simulink library "roshelperlib"  (R2024a)
settings: Solver=VariableStepAuto  StartTime=0.0  StopTime=10.0  RelTol=1e-3
values from neighbouring files (symbols this model uses):
  data = rand(prod(dims),1)    [bufferAssignTest.m]
  isVarsize = ws.get('isVarsize')    [extractmulticallbacks.m]    (also in gendatacallbacks.m = varsizeDims; rospubcallbacks.m = matlab.lang.OnOffSwitchState(commonmaskutils.getWSValue('isV; rossubcallbacks.m)
  varsize = false    [visualizeScene.m]
undefined symbols (not defined in the file or in its folder): data_SL_Info, layout, stride, x, y, z
libraries: ros2lib x4, $bdroot x2
settings Model: Creator=cstabile  LastModifiedBy=cstabile

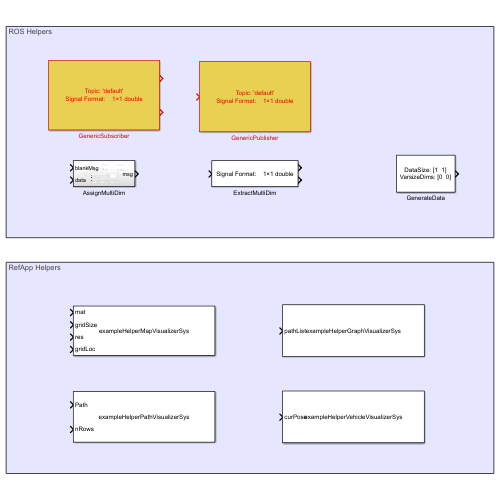
[thumbnail: Simulink's stored preview of the top-level diagram]
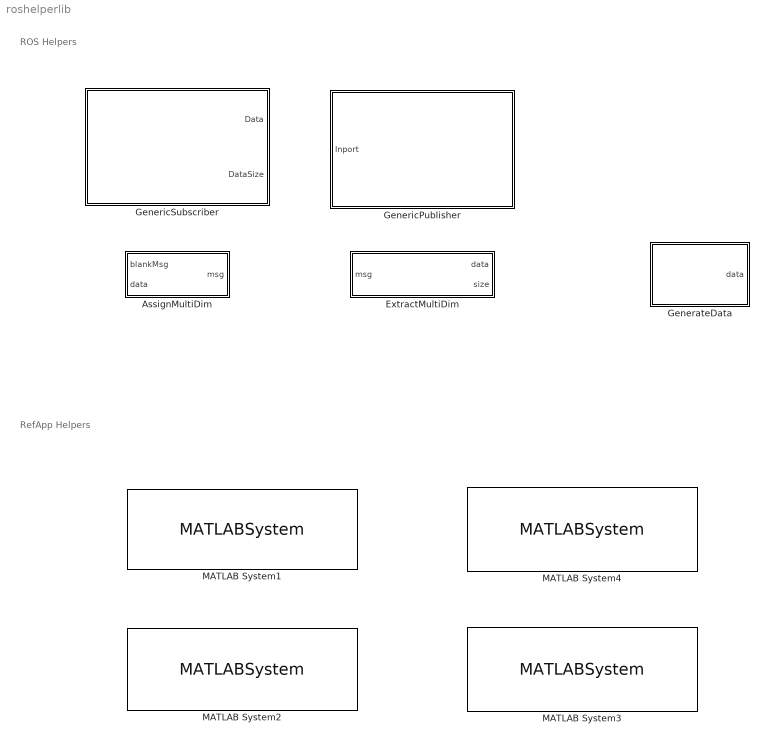
== system roshelperlib ==
  note: ROS Helpers
  note: RefApp Helpers
  AssignMultiDim : Subsystem
  ExtractMultiDim : Subsystem  mask{userDataType=double, dims=[1 1], isVarsize=off, varsizeDims=[], returnFixedTF=off}
      mask prompts: userDataType "DataType"; dims "MaxDimensions"; isVarsize "IsVarsize?"; returnFixedTF "ReturnFixed?"
      mask Display:
      | userDataType = char(get_param(gcb,'userDataType'));
      | isVarsize = matlab.lang.OnOffSwitchState(get_param(gcb,'isVarsize'));
      | dims = eval(get_param(gcb,'dims'));
      | vDims = eval(get_param(gcb,'varsizeDims'));
      | returnFixedTF = matlab.lang.OnOffSwitchState(get_param(gcb,'returnFixedTF'));
      | 
      | data = zeros(0,userDataType);
      | if isVarsize && returnFixedTF == 0 && any(vDims)
      |     type = coder.typeof(data,dims,vDims);
      | else
      |     type = coder.typeof(data,dims);
      | end
      | strs = string(splitlines(formattedDisplayText(type)));
      | dataStr = strs(2);
      | 
      | dispStrings(1) = string(['Signal Format' ': ' char(dataStr)]);
      | if isVarsize
      |     dispStrings(2) = string(['VarsizeDimensions' ': ' '[' num2str(vDims) ']']);
      | end
      | 
      | disp(dispStrings);
  GenerateData : Subsystem  mask{dataSize=[1 1], varsizeDims=[]}
      mask Display:
      | dataSize = eval(get_param(gcb,'dataSize'));
      | mask = Simulink.Mask.get(gcb);
      | vars = mask.getWorkspaceVariables;
      | isVarsize = vars(arrayfun(@(x)isequal(x.Name,'isVarsize'),vars)).Value;
      | 
      | dispStr(1) = "DataSize: " + "[" + num2str(dataSize) + "]";
      | dispStr(2) = "VarsizeDims: " + "[" + num2str(isVarsize) + "]";
      | disp(dispStr);
  GenericPublisher : Subsystem  mask{userDataType=double, dims=[1 1], topicName='default', isVarsize=off, varsizeDims=[1 0]}
      mask prompts: userDataType "Type"; dims "MaxDimension"; isVarsize "IsVarsize?"; varsizeDims "VszDims"
      mask Display:
      | userDataType = char(get_param(gcb,'userDataType'));
      | topicName = char(get_param(gcb,'topicName'));
      | isVarsize = matlab.lang.OnOffSwitchState(get_param(gcb,'isVarsize'));
      | dims = eval(get_param(gcb,'dims'));
      | vDims = eval(get_param(gcb,'varsizeDims'));
      | 
      | data = zeros(0,userDataType);
      | if isVarsize && any(vDims)
      |     type = coder.typeof(data,dims,vDims);
      | else
      |     type = coder.typeof(data,dims);
      | end
      | strs = string(splitlines(formattedDisplayText(type)));
      | dataStr = strs(2);
      | 
      | dispStrings(1) = string(['Topic' ': ' char(topicName)]);
      | dispStrings(2) = string(['Signal Format' ': ' char(dataStr)]);
      | % dispStrings(3) = string(['VarsizeDimensions' ': ' '[' num2str(vDims) ']']);
      | disp(dispStrings);
  GenericSubscriber : Subsystem  mask{userDataType=double, dims=[1 1], topicName='default', isVarsize=off, varsizeDims=[1 0], returnFixedTF=off}
      mask prompts: userDataType "Type"; dims "MaxDimension"; isVarsize "IsVarsize?"; varsizeDims "VszDims"; returnFixedTF "ReturnFixed"
      mask Display:
      | userDataType = char(get_param(gcb,'userDataType'));
      | topicName = char(get_param(gcb,'topicName'));
      | isVarsize = matlab.lang.OnOffSwitchState(get_param(gcb,'isVarsize'));
      | dims = eval(get_param(gcb,'dims'));
      | vDims = eval(get_param(gcb,'varsizeDims'));
      | returnFixedTF = matlab.lang.OnOffSwitchState(get_param(gcb,'returnFixedTF'));
      | 
      | data = zeros(0,userDataType);
      | if isVarsize && returnFixedTF == 0 && any(vDims)
      |     type = coder.typeof(data,dims,vDims);
      | else
      |     type = coder.typeof(data,dims);
      | end
      | strs = string(splitlines(formattedDisplayText(type)));
      | dataStr = strs(2);
      | 
      | dispStrings(1) = string(['Topic' ': ' char(topicName)]);
      | dispStrings(2) = string(['Signal Format' ': ' char(dataStr)]);
      | if isVarsize
      |     dispStrings(3) = string(['VarsizeDimensions' ': ' '[' num2str(vDims) ']']);
      | end
      | disp(dispStrings);
  MATLAB System1 : MATLABSystem  System=exampleHelperMapVisualizerSys  MapType=SDF  DisplayVisual=on  SimulateUsing=Interpreted execution
      mask Type: exampleHelperMapVisualizerSys
      mask Display:
      | disp('exampleHelperMapVisualizerSys');
      | port_label('input',1,'mat');
      | port_label('input',2,'gridSize');
      | port_label('input',3,'res');
      | port_label('input',4,'gridLoc');
  MATLAB System2 : MATLABSystem  System=exampleHelperPathVisualizerSys  VisualizationParameters={'k-'}  PlotType=Line  DisplayVisual=on  SimulateUsing=Interpreted execution
      mask Type: exampleHelperPathVisualizerSys
      mask Display:
      | disp('exampleHelperPathVisualizerSys');
      | port_label('input',1,'Path');
      | port_label('input',2,'nRows');
  MATLAB System3 : MATLABSystem  System=exampleHelperVehicleVisualizerSys  NumCircles=3  Length=4  Width=2  DisplayVisual=on  SimulateUsing=Interpreted execution
      mask Type: exampleHelperVehicleVisualizerSys
      mask Display:
      | disp('exampleHelperVehicleVisualizerSys');
      | port_label('input',1,'curPose');
  MATLAB System4 : MATLABSystem  System=exampleHelperGraphVisualizerSys  NodeColor=r  EdgeColor=r  LineStyle=-  GraphSpec=cell(1,0)  NetworkColor=b  NetworkStyle=:  NetworkSpec=cell(1,0)  MaxEdgeElem=Inf  NetworkAlpha=1  EdgeAlpha=1  DisplayVisual=on  SimulateUsing=Interpreted execution
      mask Type: exampleHelperGraphVisualizerSys
      mask Display:
      | disp('exampleHelperGraphVisualizerSys');
      | port_label('input',1,'pathList');

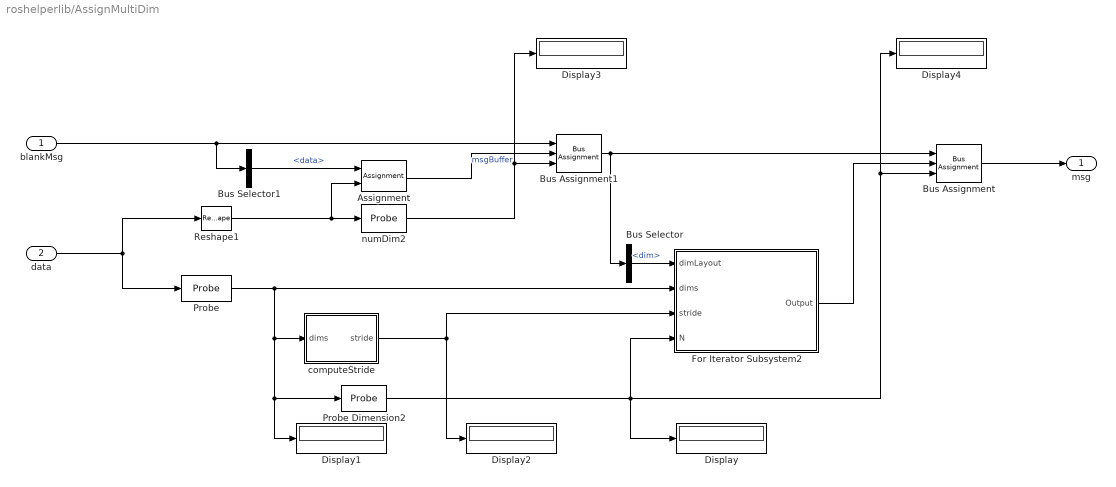
== system roshelperlib/AssignMultiDim ==
  blankMsg : Inport
  data : Inport  Port=2
  Assignment : Assignment  DiagnosticForDimensions=Warning  IndexOptions=Starting index (dialog)  Indices=1  OutputSizes=1
  Bus Assignment : BusAssignment  AssignedSignals=layout.dim,layout.dim_SL_Info.CurrentLength
  Bus Assignment1 : BusAssignment  AssignedSignals=data,data_SL_Info.CurrentLength
  Bus Selector : BusSelector  OutputSignals=layout.dim
  Bus Selector1 : BusSelector  OutputSignals=data
  Display{,1..4} (5 alike) : Display
  For Iterator Subsystem2 : Subsystem  TreatAsAtomicUnit=on
  Probe : Probe  ProbeWidth=off  ProbeSampleTime=off  ProbeComplexSignal=off  ProbeSignalDimensions=on
  Probe Dimension2 : Probe  ProbeWidth=off  ProbeSampleTime=off  ProbeComplexSignal=off  ProbeSignalDimensions=on  ProbeWidthDataType=uint32  ProbeDimensionsDataType=uint32
  Reshape1 : Reshape
  computeStride : MATLAB Function  TreatAsAtomicUnit=on
  numDim2 : Probe  ProbeSampleTime=off  ProbeComplexSignal=off  ProbeWidthDataType=uint32
  msg : Outport
  wires:
  Bus Selector1/1 -> Assignment/1  "<data>"
  Bus Selector/1 -> For Iterator Subsystem2/1(dimLayout)  "<dim>"
  Assignment/1 -> Bus Assignment1/2  "msgBuffer"
  Bus Assignment1/1 -> Bus Selector/1, Bus Assignment/1
  Probe Dimension2/1 -> For Iterator Subsystem2/4(N), Display/1, Display4/1, Bus Assignment/3
  computeStride/1(stride) -> For Iterator Subsystem2/3(stride), Display2/1
  For Iterator Subsystem2/1(Output) -> Bus Assignment/2
  blankMsg/1 -> Bus Selector1/1, Bus Assignment1/1
  Bus Assignment/1 -> msg/1
  Probe/1 -> For Iterator Subsystem2/2(dims), Probe Dimension2/1, Display1/1, computeStride/1(dims)
  numDim2/1 -> Display3/1, Bus Assignment1/3
  Reshape1/1 -> numDim2/1, Assignment/2
  data/1 -> Probe/1, Reshape1/1

== system roshelperlib/ExtractMultiDim ==
  msg : Inport
  FixedOrVarOutput : Subsystem  Variant=on  VariantControl=Subsystem
  data : Outport
  size : Outport  Port=2
  wires:
  msg/1 -> FixedOrVarOutput/1(msg)
  FixedOrVarOutput/1(data) -> data/1
  FixedOrVarOutput/2(size) -> size/1

== system roshelperlib/GenerateData ==
  Subsystem : Subsystem  Variant=on  VariantControl=Subsystem
  data : Outport
  wires:
  Subsystem/1(data) -> data/1

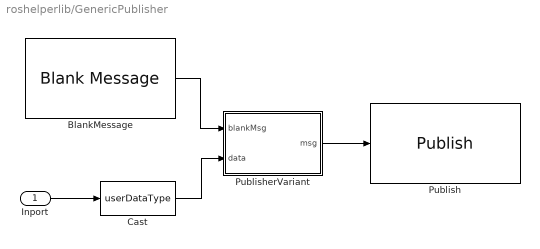
== system roshelperlib/GenericPublisher ==
  Inport : Inport
  BlankMessage : ros2lib/Blank Message  VariantControl=Choice_1  messageClass=Message  entityType=std_msgs/Float64  messageType=std_msgs/Float64  SampleTime=inf
  Cast : DataTypeConversion  OutDataTypeStr=userDataType  SaturateOnIntegerOverflow=off  RndMeth=Floor
  Publish : ros2lib/Publish  topicSource=Select from ROS network  topic=/default  messageType=std_msgs/Float64  QOSHistory=Keep last  QOSDepth=1  QOSReliability=Reliable  QOSDurability=Volatile  QOSDeadline=Inf  QOSLifespan=Inf  QOSLiveliness=Automatic  QOSLeaseDuration=Inf  QOSAvoidROSNamespaceConventions=off
  PublisherVariant : Subsystem  Variant=on  VariantControl=useFixedTF==0
  wires:
  Inport/1 -> Cast/1
  Cast/1 -> PublisherVariant/2(data)
  BlankMessage/1 -> PublisherVariant/1(blankMsg)
  PublisherVariant/1(msg) -> Publish/1

== system roshelperlib/GenericSubscriber ==
  SubscriberVariant : Subsystem  Variant=on  VariantControl=useFixedTF==0
  Data : Outport
  DataSize : Outport  Port=2
  wires:
  SubscriberVariant/2(Output1) -> DataSize/1
  SubscriberVariant/1(Output) -> Data/1

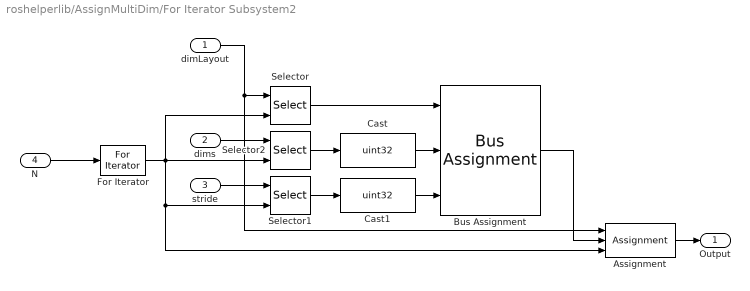
== system roshelperlib/AssignMultiDim/For Iterator Subsystem2 ==
  dimLayout : Inport
  dims : Inport  Port=2
  stride : Inport  Port=3
  N : Inport  Port=4
  Assignment : Assignment  DiagnosticForDimensions=Warning  IndexOptions=Index vector (port)  Indices=1  OutputSizes=1
  Bus Assignment : BusAssignment  AssignedSignals=size,stride
  Cast : DataTypeConversion  OutDataTypeStr=uint32  SaturateOnIntegerOverflow=off  RndMeth=Floor
  Cast1 : DataTypeConversion  OutDataTypeStr=uint32  SaturateOnIntegerOverflow=off  RndMeth=Floor
  For Iterator : ForIterator  IterationSource=external  IterationLimit=16
  Selector : Selector  InputPortWidth=16  IndexOptions=Index vector (port)  Indices=[1 3]  OutputSizes=1
  Selector1 : Selector  IndexOptions=Index vector (port)  Indices=[1 3]  OutputSizes=1
  Selector2 : Selector  IndexOptions=Index vector (port)  Indices=[1 3]  OutputSizes=1
  Output : Outport
  wires:
  stride/1 -> Selector1/1
  dims/1 -> Selector2/1
  Bus Assignment/1 -> Assignment/2
  dimLayout/1 -> Assignment/1, Selector/1
  Selector/1 -> Bus Assignment/1
  For Iterator/1 -> Selector2/2, Selector1/2, Assignment/3, Selector/2
  N/1 -> For Iterator/1
  Selector1/1 -> Cast1/1
  Selector2/1 -> Cast/1
  Assignment/1 -> Output/1
  Cast/1 -> Bus Assignment/2
  Cast1/1 -> Bus Assignment/3

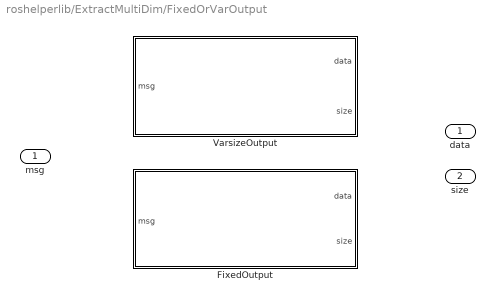
== system roshelperlib/ExtractMultiDim/FixedOrVarOutput ==
  msg : Inport
  FixedOutput : Subsystem  VariantControl=outputIsFixedTF==1
  VarsizeOutput : Subsystem  VariantControl=outputIsFixedTF==0
  data : Outport
  size : Outport  Port=2

== system roshelperlib/GenerateData/Subsystem ==
  Fixed : Subsystem  VariantControl=variantFixedTF == 1
  Varsize : Subsystem  VariantControl=variantFixedTF == 0
  data : Outport

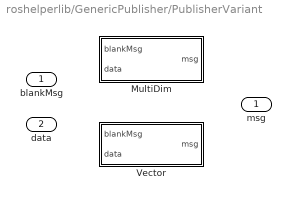
== system roshelperlib/GenericPublisher/PublisherVariant ==
  blankMsg : Inport
  data : Inport  Port=2
  MultiDim : Subsystem  VariantControl=useVarsizeTF==1
  Vector : Subsystem  VariantControl=useVarsizeTF==0
  msg : Outport

== system roshelperlib/GenericSubscriber/SubscriberVariant ==
  MultiDim : Subsystem  VariantControl=useMultiDimTF==1
  Vector : Subsystem  VariantControl=useMultiDimTF==0
  Output : Outport
  Output1 : Outport  Port=2

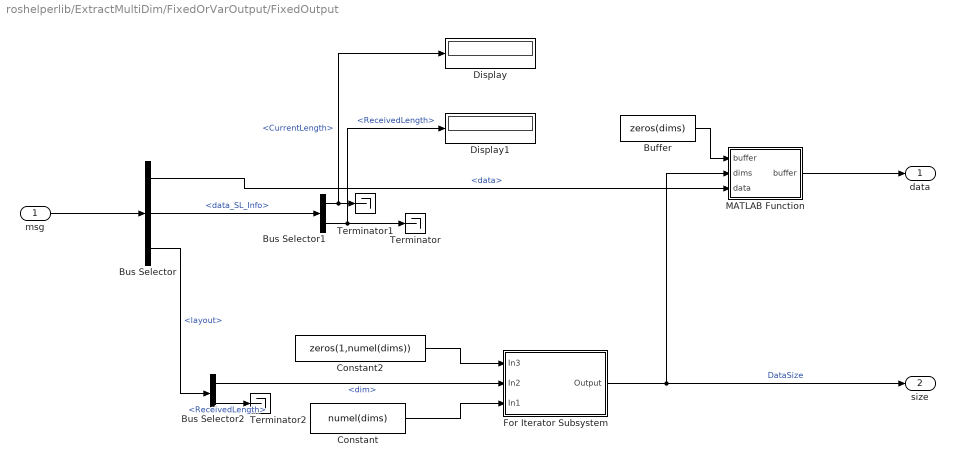
== system roshelperlib/ExtractMultiDim/FixedOrVarOutput/FixedOutput ==
  msg : Inport
  Buffer : Constant  Value=zeros(dims)  OutDataTypeStr=userDataType
  Bus Selector : BusSelector  OutputSignals=data,data_SL_Info,layout
  Bus Selector1 : BusSelector  OutputSignals=CurrentLength,ReceivedLength
  Bus Selector2 : BusSelector  OutputSignals=dim,dim_SL_Info.ReceivedLength
  Constant : Constant  Value=numel(dims)
  Constant2 : Constant  Value=zeros(1,numel(dims))  VectorParams1D=off
  Display : Display
  Display1 : Display
  For Iterator Subsystem : Subsystem  TreatAsAtomicUnit=on
  MATLAB Function : MATLAB Function  TreatAsAtomicUnit=on
  Terminator : Terminator
  Terminator1 : Terminator
  Terminator2 : Terminator
  data : Outport
  size : Outport  Port=2
  wires:
  Bus Selector/1 -> MATLAB Function/3(data)  "<data>"
  Bus Selector2/1 -> For Iterator Subsystem/2(In2)  "<dim>"
  For Iterator Subsystem/1(Output) -> MATLAB Function/2(dims), size/1  "DataSize"
  Bus Selector/3 -> Bus Selector2/1  "<layout>"
  Bus Selector2/2 -> Terminator2/1  "<ReceivedLength>"
  Bus Selector1/2 -> Terminator/1, Display1/1  "<ReceivedLength>"
  Bus Selector1/1 -> Terminator1/1, Display/1  "<CurrentLength>"
  MATLAB Function/1(buffer) -> data/1
  Buffer/1 -> MATLAB Function/1("buffer ")
  Constant2/1 -> For Iterator Subsystem/1(In3)
  Bus Selector/2 -> Bus Selector1/1  "<data_SL_Info>"
  msg/1 -> Bus Selector/1
  Constant/1 -> For Iterator Subsystem/3(In1)

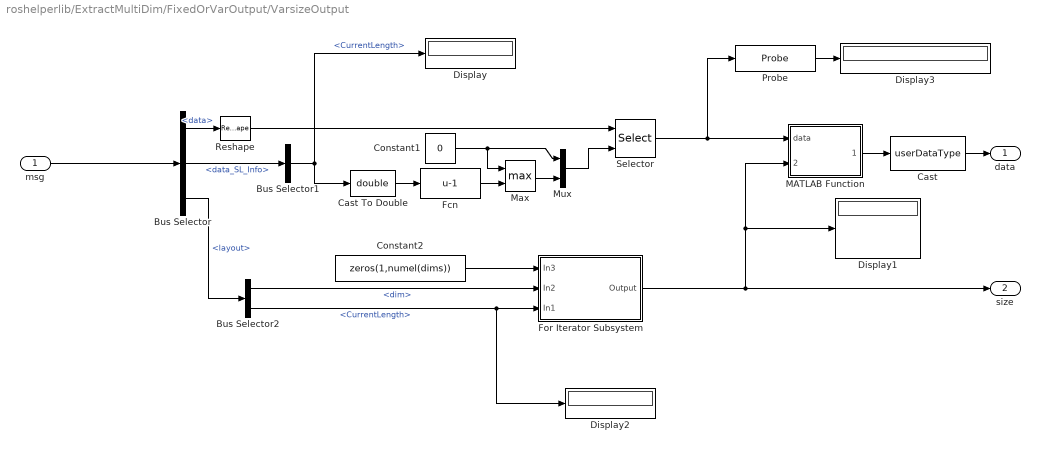
== system roshelperlib/ExtractMultiDim/FixedOrVarOutput/VarsizeOutput ==
  msg : Inport
  Bus Selector : BusSelector  OutputSignals=data,data_SL_Info,layout
  Bus Selector1 : BusSelector  OutputSignals=CurrentLength
  Bus Selector2 : BusSelector  OutputSignals=dim,dim_SL_Info.CurrentLength
  Cast : DataTypeConversion  OutDataTypeStr=userDataType  SaturateOnIntegerOverflow=off  RndMeth=Floor
  Cast To Double : DataTypeConversion  OutDataTypeStr=double  SaturateOnIntegerOverflow=off  RndMeth=Floor
  Constant1 : Constant  Value=0
  Constant2 : Constant  Value=zeros(1,numel(dims))  VectorParams1D=off
  Display{,1..3} (4 alike) : Display
  Fcn : Fcn  Expr=u-1
  For Iterator Subsystem : Subsystem  TreatAsAtomicUnit=on
  MATLAB Function : MATLAB Function  TreatAsAtomicUnit=on
  Max : MinMax  Function=max  Inputs=2
  Mux : Mux  Inputs=2
  Probe : Probe  ProbeWidth=off  ProbeSampleTime=off  ProbeComplexSignal=off  ProbeSignalDimensions=on
  Reshape : Reshape  OutputDimensionality=Column vector (2-D)
  Selector : Selector  NumberOfDimensions=2  IndexMode=Zero-based  InputPortWidth=1  IndexOptions=Starting and ending indices (port),Select all  Indices=[1 3],1  OutputSizes=1,1
  data : Outport
  size : Outport  Port=2
  wires:
  Constant2/1 -> For Iterator Subsystem/1(In3)
  Bus Selector/3 -> Bus Selector2/1  "<layout>"
  Bus Selector1/1 -> Cast To Double/1, Display/1  "<CurrentLength>"
  Bus Selector/1 -> Reshape/1  "<data>"
  MATLAB Function/1(reshapedData) -> Cast/1
  For Iterator Subsystem/1(Output) -> size/1, Display1/1, MATLAB Function/2(receiveDims)
  Mux/1 -> Selector/2
  Selector/1 -> Probe/1, MATLAB Function/1(data)
  Constant1/1 -> Mux/1, Max/1
  Bus Selector2/1 -> For Iterator Subsystem/2(In2)  "<dim>"
  Cast To Double/1 -> Fcn/1
  Bus Selector/2 -> Bus Selector1/1  "<data_SL_Info>"
  Bus Selector2/2 -> For Iterator Subsystem/3(In1), Display2/1  "<CurrentLength>"
  msg/1 -> Bus Selector/1
  Cast/1 -> data/1
  Reshape/1 -> Selector/1
  Max/1 -> Mux/2
  Fcn/1 -> Max/2
  Probe/1 -> Display3/1

== system roshelperlib/GenerateData/Subsystem/Fixed ==
  Constant : Constant  Value=rand(dataSize)
  data : Outport
  wires:
  Constant/1 -> data/1

== system roshelperlib/GenerateData/Subsystem/Varsize ==
  MATLAB Function1 : MATLAB Function  TreatAsAtomicUnit=on
  data : Outport
  wires:
  MATLAB Function1/1(data) -> data/1

== system roshelperlib/GenericPublisher/PublisherVariant/MultiDim ==
  blankMsg : Inport
  data : Inport  Port=2
  AssignMultiDim : $bdroot/AssignMultiDim  SystemSampleTime=-1  VariantActivationTime=update diagram  AllowFlexibleInterface=on  Latency=0  AutoFrameSizeCalculation=off
  msg : Outport
  wires:
  data/1 -> AssignMultiDim/2
  blankMsg/1 -> AssignMultiDim/1
  AssignMultiDim/1 -> msg/1

== system roshelperlib/GenericPublisher/PublisherVariant/Vector ==
  blankMsg : Inport
  data : Inport  Port=2
  Subsystem : Subsystem  Variant=on  VariantControl=Subsystem
  msg : Outport
  wires:
  data/1 -> Subsystem/2(data)
  blankMsg/1 -> Subsystem/1(blankMsg)
  Subsystem/1(msg) -> msg/1

== system roshelperlib/GenericSubscriber/SubscriberVariant/MultiDim ==
  Subscribe : ros2lib/Subscribe  topicSource=Specify your own  topic=/varsize  messageType=std_msgs/Float64MultiArray  sampleTime=-1  QOSHistory=Keep last  QOSDepth=1  QOSReliability=Reliable  QOSDurability=Volatile  QOSDeadline=Inf  QOSLifespan=Inf  QOSLiveliness=Automatic  QOSLeaseDuration=Inf  QOSAvoidROSNamespaceConventions=off
  Subsystem : Subsystem
  Output : Outport
  Output1 : Outport  Port=2
  wires:
  Subsystem/2(size) -> Output1/1
  Subsystem/1(data) -> Output/1
  Subscribe/1 -> Subsystem/Enable
  Subscribe/2 -> Subsystem/1(msg)

== system roshelperlib/GenericSubscriber/SubscriberVariant/Vector ==
  Subscribe : ros2lib/Subscribe  topicSource=Specify your own  topic=/default  messageType=std_msgs/Float64  sampleTime=-1  QOSHistory=Keep last  QOSDepth=1  QOSReliability=Reliable  QOSDurability=Volatile  QOSDeadline=Inf  QOSLifespan=Inf  QOSLiveliness=Automatic  QOSLeaseDuration=Inf  QOSAvoidROSNamespaceConventions=off
  Subsystem : Subsystem
  Output : Outport
  Output1 : Outport  Port=2
  wires:
  Subsystem/2(Out2) -> Output1/1
  Subsystem/1(Out1) -> Output/1
  Subscribe/2 -> Subsystem/1(msg)
  Subscribe/1 -> Subsystem/Enable

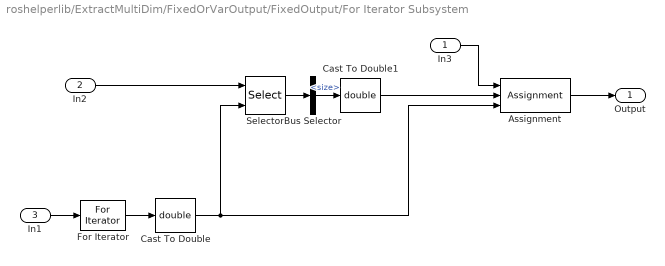
== system roshelperlib/ExtractMultiDim/FixedOrVarOutput/FixedOutput/For Iterator Subsystem ==
  In3 : Inport
  In2 : Inport  Port=2
  In1 : Inport  Port=3
  Assignment : Assignment  DiagnosticForDimensions=Warning  IndexOptions=Starting index (port)  Indices=1  OutputSizes=1
  Bus Selector : BusSelector  OutputSignals=size
  Cast To Double : DataTypeConversion  OutDataTypeStr=double  SaturateOnIntegerOverflow=off  RndMeth=Floor
  Cast To Double1 : DataTypeConversion  OutDataTypeStr=double  SaturateOnIntegerOverflow=off  RndMeth=Floor
  For Iterator : ForIterator  IterationSource=external
  Selector : Selector  InputPortWidth=16  IndexOptions=Index vector (port)  Indices=[1 3]  OutputSizes=1
  Output : Outport
  wires:
  Cast To Double1/1 -> Assignment/2
  Cast To Double/1 -> Assignment/3, Selector/2
  Assignment/1 -> Output/1
  In3/1 -> Assignment/1
  For Iterator/1 -> Cast To Double/1
  Selector/1 -> Bus Selector/1
  In2/1 -> Selector/1
  Bus Selector/1 -> Cast To Double1/1  "<size>"
  In1/1 -> For Iterator/1

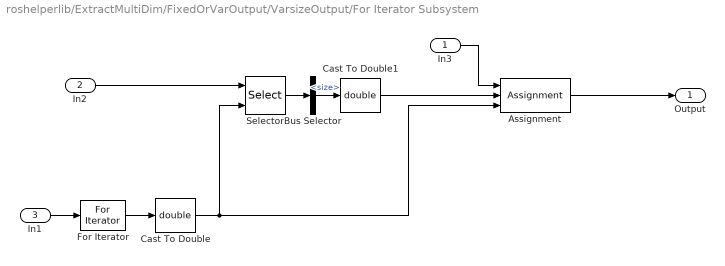
== system roshelperlib/ExtractMultiDim/FixedOrVarOutput/VarsizeOutput/For Iterator Subsystem ==
  In3 : Inport
  In2 : Inport  Port=2
  In1 : Inport  Port=3
  Assignment : Assignment  DiagnosticForDimensions=Warning  IndexOptions=Starting index (port)  Indices=1  OutputSizes=1
  Bus Selector : BusSelector  OutputSignals=size
  Cast To Double : DataTypeConversion  OutDataTypeStr=double  SaturateOnIntegerOverflow=off  RndMeth=Floor
  Cast To Double1 : DataTypeConversion  OutDataTypeStr=double  SaturateOnIntegerOverflow=off  RndMeth=Floor
  For Iterator : ForIterator  IterationSource=external
  Selector : Selector  InputPortWidth=16  IndexOptions=Index vector (port)  Indices=[1 3]  OutputSizes=1
  Output : Outport
  wires:
  Cast To Double/1 -> Assignment/3, Selector/2
  Cast To Double1/1 -> Assignment/2
  Assignment/1 -> Output/1
  In3/1 -> Assignment/1
  For Iterator/1 -> Cast To Double/1
  Selector/1 -> Bus Selector/1
  In2/1 -> Selector/1
  Bus Selector/1 -> Cast To Double1/1  "<size>"
  In1/1 -> For Iterator/1

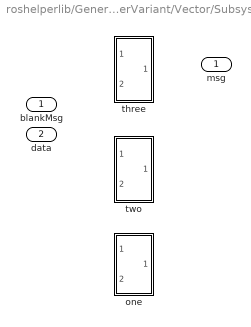
== system roshelperlib/GenericPublisher/PublisherVariant/Vector/Subsystem ==
  blankMsg : Inport
  data : Inport  Port=2
  one : Subsystem  VariantControl=N==1
  three : Subsystem  VariantControl=N==3
  two : Subsystem  VariantControl=N==2
  msg : Outport

== system roshelperlib/GenericSubscriber/SubscriberVariant/MultiDim/Subsystem ==
  msg : Inport
  Enable : EnablePort  PropagateVarSize=During execution
  FixedOrVarOutput : $bdroot/ExtractMultiDim/FixedOrVarOutput  SystemSampleTime=-1  VariantControl=Subsystem  VariantActivationTime=update diagram  AllowFlexibleInterface=on  Latency=0  AutoFrameSizeCalculation=off
      link override FixedOutput: VariantControl=outputIsFixedTF==1
      link override VarsizeOutput: VariantControl=outputIsFixedTF==0
  data : Outport
  size : Outport  Port=2
  wires:
  FixedOrVarOutput/1 -> data/1
  FixedOrVarOutput/2 -> size/1
  msg/1 -> FixedOrVarOutput/1

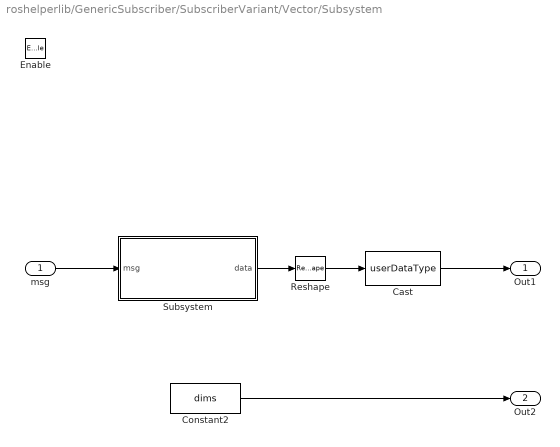
== system roshelperlib/GenericSubscriber/SubscriberVariant/Vector/Subsystem ==
  msg : Inport
  Enable : EnablePort  PropagateVarSize=During execution
  Cast : DataTypeConversion  OutDataTypeStr=userDataType  SaturateOnIntegerOverflow=off  RndMeth=Floor
  Constant2 : Constant  Value=dims
  Reshape : Reshape  OutputDimensionality=Customize  OutputDimensions=dims
  Subsystem : Subsystem  Variant=on  VariantControl=Subsystem
  Out1 : Outport
  Out2 : Outport  Port=2
  wires:
  Constant2/1 -> Out2/1
  Subsystem/1(data) -> Reshape/1
  Cast/1 -> Out1/1
  msg/1 -> Subsystem/1(msg)
  Reshape/1 -> Cast/1

== system roshelperlib/GenericPublisher/PublisherVariant/Vector/Subsystem/one ==
  blankMsg : Inport
  data : Inport  Port=2
  Bus Assignment : BusAssignment  AssignedSignals=data
  Cast : DataTypeConversion  OutDataTypeStr=userDataType  SaturateOnIntegerOverflow=off  RndMeth=Floor
  msg : Outport
  wires:
  blankMsg/1 -> Bus Assignment/1
  data/1 -> Cast/1
  Bus Assignment/1 -> msg/1
  Cast/1 -> Bus Assignment/2

== system roshelperlib/GenericPublisher/PublisherVariant/Vector/Subsystem/three ==
  blankMsg : Inport
  data : Inport  Port=2
  Bus Assignment : BusAssignment  AssignedSignals=x,y,z
  Demux : Demux  Outputs=3
  msg : Outport
  wires:
  blankMsg/1 -> Bus Assignment/1
  Bus Assignment/1 -> msg/1
  data/1 -> Demux/1
  Demux/3 -> Bus Assignment/4
  Demux/2 -> Bus Assignment/3
  Demux/1 -> Bus Assignment/2

== system roshelperlib/GenericPublisher/PublisherVariant/Vector/Subsystem/two ==
  blankMsg : Inport
  data : Inport  Port=2
  Bus Assignment : BusAssignment  AssignedSignals=x,y
  Demux : Demux  Outputs=2
  msg : Outport
  wires:
  data/1 -> Demux/1
  blankMsg/1 -> Bus Assignment/1
  Demux/2 -> Bus Assignment/3
  Bus Assignment/1 -> msg/1
  Demux/1 -> Bus Assignment/2

== system roshelperlib/GenericSubscriber/SubscriberVariant/Vector/Subsystem/Subsystem ==
  msg : Inport
  one : Subsystem  VariantControl=N==1
  three : Subsystem  VariantControl=N==3
  two : Subsystem  VariantControl=N==2
  data : Outport

== system roshelperlib/GenericSubscriber/SubscriberVariant/Vector/Subsystem/Subsystem/one ==
  msg : Inport
  Bus Selector : BusSelector  OutputSignals=data
  data : Outport
  wires:
  msg/1 -> Bus Selector/1
  Bus Selector/1 -> data/1  "<data>"

== system roshelperlib/GenericSubscriber/SubscriberVariant/Vector/Subsystem/Subsystem/three ==
  msg : Inport
  Bus Selector : BusSelector  OutputSignals=x,y,z
  Mux : Mux  Inputs=3
  data : Outport
  wires:
  msg/1 -> Bus Selector/1
  Mux/1 -> data/1
  Bus Selector/1 -> Mux/1  "<x>"
  Bus Selector/2 -> Mux/2  "<y>"
  Bus Selector/3 -> Mux/3  "<z>"

== system roshelperlib/GenericSubscriber/SubscriberVariant/Vector/Subsystem/Subsystem/two ==
  msg : Inport
  Bus Selector : BusSelector  OutputSignals=x,y
  Mux : Mux  Inputs=2
  data : Outport
  wires:
  msg/1 -> Bus Selector/1
  Mux/1 -> data/1
  Bus Selector/2 -> Mux/2  "<y>"
  Bus Selector/1 -> Mux/1  "<x>"

== matlab function roshelperlib/AssignMultiDim/computeStride ==
  data: dims input; stride output
function stride = fcn(dims)
    stride = cumprod([1 dims(1:end-1)']);

== matlab function roshelperlib/GenerateData/Subsystem/Varsize/MATLAB Function1 ==
  data: data output size=dataSize; dataSize parameter; isVarsize parameter
function data = generateVarsizeData(dataSize, isVarsize)
    n = numel(dataSize);
    sz = dataSize;
    for i = 1:n
        if isVarsize(i)
            sz(i) = randi([1,dataSize(i)],1);
        end
    end
    data = rand(sz);
end

== matlab function roshelperlib/ExtractMultiDim/FixedOrVarOutput/VarsizeOutput/MATLAB Function ==
  data: data input; receiveDims input size=[1 numel(dims)]; reshapedData output size=dims
function reshapedData = makeVarsize(data, receiveDims)
reshapedData = zeros(receiveDims,'like',data);
if prod(receiveDims) ~= 0
    reshapedData(:) = data(1:prod(receiveDims),1);
end

== matlab function roshelperlib/ExtractMultiDim/FixedOrVarOutput/FixedOutput/MATLAB Function ==
  data: buffer input; dims input; data input; buffer output
function buffer = fcn(buffer, dims, data)
    buffer = subassignBuffer(buffer,dims,data(1:prod(dims)));
end
